simulink model "day07_vehicle_speed_feedback"  (R2026a)
settings: Solver=VariableStepAuto  StopTime=25
libraries: simulink x3
settings Model: Creator=DELL  LastModifiedBy=DELL

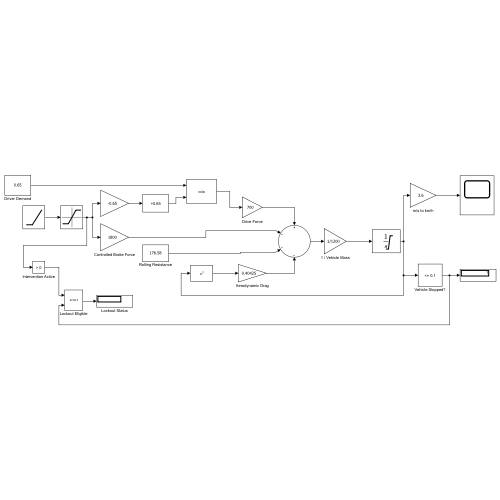
[thumbnail: Simulink's stored preview of the top-level diagram]
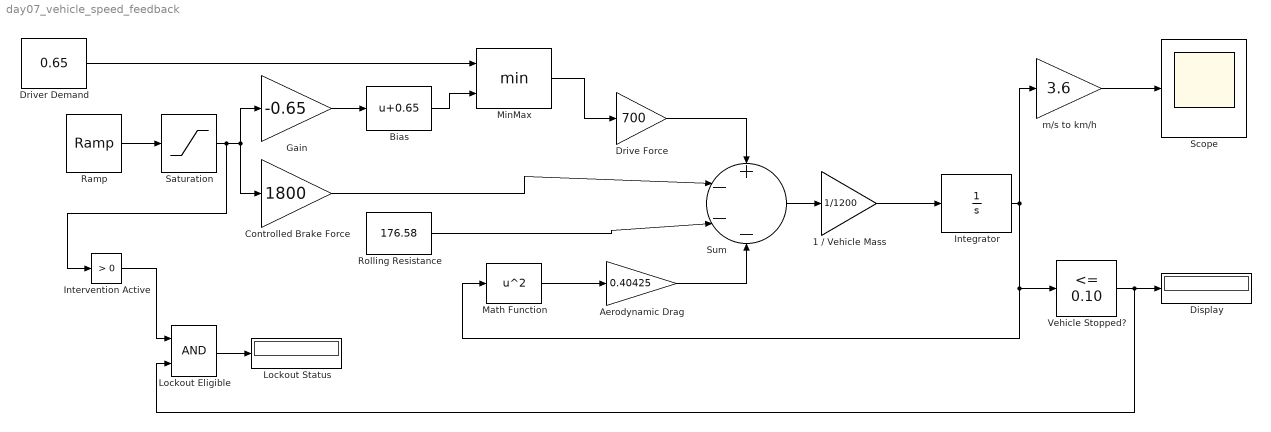
== system day07_vehicle_speed_feedback ==
  1 / Vehicle Mass : Gain  Gain=1/1200
  Aerodynamic Drag : Gain  Gain=0.40425
  Bias : Bias  Bias=0.65  SaturateOnIntegerOverflow=off
  Controlled Brake Force : Gain  Gain=1800
  Display : Display
  Drive Force : Gain  Gain=700
  Driver Demand : Constant  Value=0.65
  Gain : Gain  Gain=-0.65
  Integrator : Integrator  InitialCondition=20  LimitOutput=on  LowerSaturationLimit=0  ZeroCross=off
  Intervention Active : simulink/Logic and Bit Operations/Compare To Constant  relop=>  const=0  OutDataTypeStr=boolean
  Lockout Eligible : Logic  AllPortsSameDT=off  OutDataTypeStr=boolean
  Lockout Status : Display
  Math Function : Math  Operator=square
  MinMax : MinMax  Inputs=2
  Ramp : simulink/Sources/Ramp  slope=1/6  start=5  InitialOutput=0
  Rolling Resistance : Constant  Value=176.58
  Saturation : Saturate  UpperLimit=1  LowerLimit=0
  Scope : Scope
      settings: ActiveDisplayYMinimum=-9.2143800531365976  ActiveDisplayYMaximum=82.929420478229389
  Sum : Sum  Inputs=+---
  Vehicle Stopped? : simulink/Logic and Bit Operations/Compare To Constant  relop=<=  const=0.10  OutDataTypeStr=boolean
  m/s to km/h : Gain  Gain=3.6
  wires:
  Driver Demand/1 -> MinMax/1
  Ramp/1 -> Saturation/1
  Saturation/1 -> Intervention Active/1, Gain/1, Controlled Brake Force/1
  Gain/1 -> Bias/1
  Bias/1 -> MinMax/2
  MinMax/1 -> Drive Force/1
  Drive Force/1 -> Sum/1
  Controlled Brake Force/1 -> Sum/2
  Rolling Resistance/1 -> Sum/3
  Sum/1 -> 1 / Vehicle Mass/1
  1 / Vehicle Mass/1 -> Integrator/1
  Integrator/1 -> m/s to km/h/1, Vehicle Stopped?/1, Math Function/1
  m/s to km/h/1 -> Scope/1
  Math Function/1 -> Aerodynamic Drag/1
  Aerodynamic Drag/1 -> Sum/4
  Vehicle Stopped?/1 -> Lockout Eligible/2, Display/1
  Intervention Active/1 -> Lockout Eligible/1
  Lockout Eligible/1 -> Lockout Status/1
